simulink model "SimplePendulumWithFeedback"  (Simulink 8.3)
settings: Solver=ode45  StartTime=0.0  StopTime=T  RelTol=1e-3
values from neighbouring files (symbols this model uses):
  b = bsy0s(i, 1)    [chapter2.m]    (also in pendulum1.m = 0; pendulum2.m = 0; pendulum3.m = 0; pendulum4.m = 0)
  den = conv([1 -pp(1)], [1 -pp(2)])    [pendulum1.m]    (also in pendulum2.m = Gpi.den{1}; pendulum4.m = ctr.den{1})
  g = tf(pOverMHat,[1 bOverMHat])    [chapter2.m]    (also in chapter4.m = tf(pOverMHat, [1 bOverMHat]); pendulum1.m = 9.8; pendulum2.m = 9.8; pendulum3.m = 9.8)
  Jr = (J+m*r^2)    (= 0.015)    [pendulum1.m]    (also in pendulum2.m; pendulum3.m; pendulum4.m)
  m = length(z) - 1    [basym.m]    (also in pendulum1.m = 0.5; pendulum2.m = 0.5; pendulum3.m = 0.5; pendulum4.m = 0.5)
  num = ctr.num{1}    [pendulum4.m]
  r = r(1 : Nlambda)    [chapter2.m]    (also in chapter6.m = {}; pendulum1.m = 0.15; pendulum2.m = 0.15; pendulum3.m = 0.15)
  theta0 = y1{i}(end)    [pendulum4.m]
  thetaBar = atan(.1)    [chapter2.m]    (also in chapter4.m; pendulum4.m = 2.35619449019)
settings Model: Creator=mauricio  LastModifiedBy=mauricio
settings OptimizationCC: ExpressionDepthLimit=2147483647
settings DebuggingCC: SolverPrmCheckMsg=none  FcnCallInpInsideContextMsg=UseLocalSettings

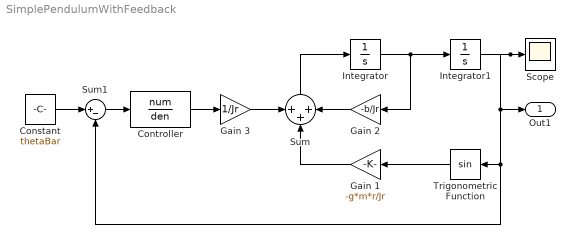
== system SimplePendulumWithFeedback ==
  Constant : Constant  Value=thetaBar
  Controller : TransferFcn  Numerator=num  Denominator=den
  Gain 1 : Gain  Gain=-g*m*r/Jr
  Gain 2 : Gain  Gain=-b/Jr
  Gain 3 : Gain  Gain=1/Jr
  Integrator : Integrator
  Integrator1 : Integrator  InitialCondition=theta0
  Scope : Scope
      settings: YMin=-3.141592653589793  YMax=3.141592653589793
  Sum : Sum  Inputs=+++
  Sum1 : Sum  Inputs=|+-
  Trigonometric Function : Trigonometry
  Out1 : Outport
  wires:
  Integrator/1 -> Integrator1/1, Gain 2/1
  Integrator1/1 -> Scope/1, Trigonometric Function/1, Sum1/2, Out1/1
  Trigonometric Function/1 -> Gain 1/1
  Sum/1 -> Integrator/1
  Gain 2/1 -> Sum/3
  Gain 1/1 -> Sum/2
  Sum1/1 -> Controller/1
  Controller/1 -> Gain 3/1
  Constant/1 -> Sum1/1
  Gain 3/1 -> Sum/1
